simulink model "rtwdemo_asap2"  (Simulink 6.0)
settings: Solver=FixedStepDiscrete  StartTime=0.0  StopTime=10.0  RelTol=1e-3
PostLoadFcn:
  | rtwdemo_asap2_data
values from neighbouring files (symbols this model uses):
  k1 = Simulink.Parameter    [rtwdemo_asap2_data.m]    (also in rtwdemo_reusable_data.m)
  k2 = Simulink.Parameter    [rtwdemo_asap2_data.m]
  xbreak1 = Simulink.Parameter    [rtwdemo_asap2_data.m]
  ydata = Simulink.Parameter    [rtwdemo_asap2_data.m]
  zdata = Simulink.Parameter    [rtwdemo_asap2_data.m]
libraries: rtwdemowidgets x3
settings Model: Creator=The MathWorks Inc.  LastModifiedBy=batserve  ExtModeAutoUpdateStatusClock=off  TunableVars=K_ExpGlob,K_ExpGlob_FixPt,K_ImpExt,K_ImpExtPt,K_ImpExtPt_FixPt,K_ImpExt_FixPt,K_SimGlob,K_SimGlob_FixPt,XBreak,XBreak_FixPt,YBreak,YBreak_FixPt,YData_ExpGlob,YData_ExpGlob_FixPt,YData_ImpExt,YData_ImpExtPt,YData_ImpExtPt_FixPt,YData_ImpExt_FixPt,YData_SimGlob,YData_SimGlob_FixPt,ZData_ExpGlob,ZData_ExpGlob_FixPt,ZData_ImpExt,ZData_ImpExtPt,ZData_ImpExtPt_FixPt,ZData_ImpExt_FixPt,ZData_SimGlob,ZData_SimGlob_FixPt  TunableVarsStorageClass=ExportedGlobal,ExportedGlobal,ImportedExtern,ImportedExternPointer,ImportedExternPointer,ImportedExtern,Auto,Auto,ExportedGlobal,ExportedGlobal,ExportedGlobal,ExportedGlobal,ExportedGlobal,ExportedGlobal,ImportedExtern,ImportedExternPointer,ImportedExternPointer,ImportedExtern,Auto,Auto,ExportedGlobal,ExportedGlobal,ImportedExtern,ImportedExternPointer,ImportedExternPointer,ImportedExtern,Auto,Auto  TunableVarsTypeQualifier=,,,,,,,,,,,,,,,,,,,,,,,,,,,
settings DataIOCC: SaveOutput=off  SaveTime=off  SignalLoggingName=sigsOut
settings OptimizationCC: InlineParams=on  EnforceIntegerDowncast=off  StateBitsets=on  DataBitsets=on  UseTempVars=on
settings DebuggingCC: CheckExecutionContextPreStartOutputMsg=on  CheckExecutionContextRuntimeOutputMsg=on  SignalResolutionControl=TryResolveAll  SolverPrmCheckMsg=none
settings RTWCC: TLCOptions=-p0 -aWarnNonSaturatedBlocks=0  GenCodeOnly=on  GenerateReport=on  RTWVerbose=off  ProcessScript=grt_make_rtw_hook  LaunchReport=on
settings CodeAppCC: ForceParamTrailComments=on  PrefixModelToSubsysFcnNames=off
settings GRTTargetCC: MatFileLogging=off  GenerateASAP2=on

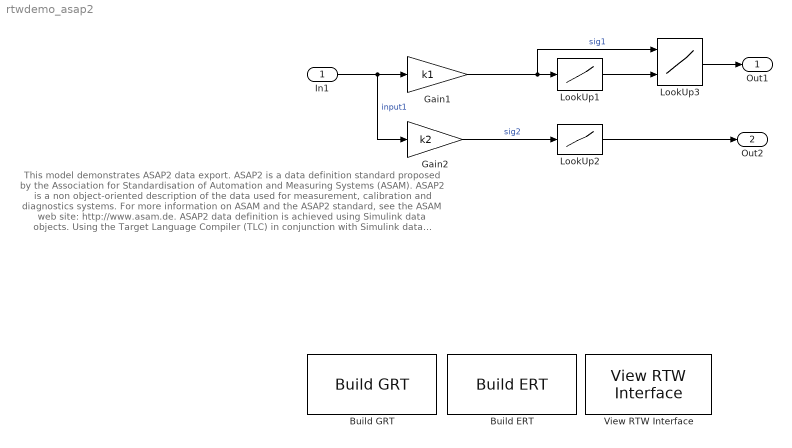
== system rtwdemo_asap2 ==
  note: This model demonstrates ASAP2 data export.  ASAP2 is a data definition standard proposed by the
      | Association for Standardisation of Automation and Measuring Systems (ASAM). ASAP2 is a non
      | object-oriented description of the data used for measurement, calibration and diagnostics systems.  For
      | more information on ASAM and the ASAP2 standard, see the ASAM web site: http://www.asam.de.  ASAP2
      | data definition is achieved using Simulink data objects.  Using the Target Language Compiler (TLC) in
      | conjunction with Simulink data objects, you can create highly customized solutions for your application.
      | See the Real-Time Workshop User's Guide for complete details on ASAP2 file generation.
      |
      | You configure ASAP2 file generation from the Configuration Parameters RTW Interface page.
  In1 : Inport  Port=1  LatchInput=off
  Build ERT : rtwdemowidgets/Build ERT  attrib_overrides={'GenerateASAP2'}
  Build GRT : rtwdemowidgets/Build GRT  attrib_overrides={'GenerateASAP2'}
  Gain1 : Gain  Gain=k1  SaturateOnIntegerOverflow=on
  Gain2 : Gain  Gain=k2  SaturateOnIntegerOverflow=on
  LookUp1 : Lookup  DialogController=Simulink.DDGSource  InputValues=xbreak1  OutputValues=ydata  SaturateOnIntegerOverflow=on
  LookUp2 : Lookup  DialogController=Simulink.DDGSource  InputValues=xbreak1  OutputValues=ydata  SaturateOnIntegerOverflow=on
  LookUp3 : Lookup2D  DialogController=Simulink.DDGSource  RowIndex=xbreak2  ColumnIndex=ybreak  OutputValues=zdata  OutScaling=2^-10  InputSameDT=on
  View RTW Interface : rtwdemowidgets/View RTW Interface
  Out1 : Outport
  Out2 : Outport  Port=2
  wires:
  Gain2/1 -> LookUp2/1  "sig2"
  Gain1/1 -> LookUp1/1, LookUp3/1  "sig1"
  LookUp1/1 -> LookUp3/2
  LookUp3/1 -> Out1/1
  LookUp2/1 -> Out2/1
  In1/1 -> Gain1/1, Gain2/1  "input1"
